simulink model "ProposedProblem1"  (R2013a)
settings: Solver=ode45  StartTime=0.0  StopTime=10.0  RelTol=1e-3
undefined symbols (not defined in the file): des, gcbh
settings Model: Creator=gabig  LastModifiedBy=gabig

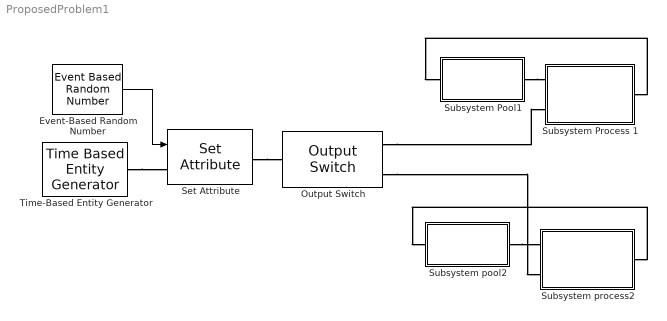
== system ProposedProblem1 ==
  Event-Based Random Number : EventBasedRandomNumber  Distribution=Arbitrary discrete  valueVecDisc=[1 2]  probVecDisc=[0.4 0.6]  Seed=12346
  Output Switch : OutputSwitch  NumberOutputPorts=2  SwitchingCriterion=From attribute  AttributeName=Type
  Set Attribute : SetAttribute  AttributeName=Type  AttributeFrom=Signal port  EvaluatedAttributeValue={ []}
  Subsystem Pool1 : Subsystem
  "Subsystem Process 1 " : Subsystem
  "Subsystem pool2 " : Subsystem
  "Subsystem process2 " : Subsystem
  Time-Based Entity Generator : TimeBasedEntityGenerator  Distribution=Uniform  Minimum=0.01  Maximum=0.2
  wires:
  Event-Based Random Number/1 -> Set Attribute/1
  connections:
  "Subsystem process2 "/RConn1 -- "Subsystem pool2 "/LConn1
  Time-Based Entity Generator/RConn1 -- Set Attribute/LConn1
  "Subsystem pool2 "/RConn1 -- "Subsystem process2 "/LConn1
  Output Switch/RConn2 -- "Subsystem process2 "/LConn2
  "Subsystem Process 1 "/RConn1 -- Subsystem Pool1/LConn1
  Output Switch/RConn1 -- "Subsystem Process 1 "/LConn2
  Set Attribute/RConn1 -- Output Switch/LConn1
  Subsystem Pool1/RConn1 -- "Subsystem Process 1 "/LConn1

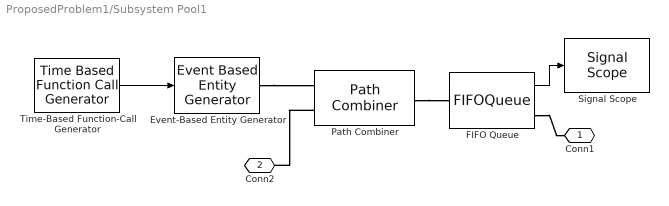
== system ProposedProblem1/Subsystem Pool1 ==
  Event-Based Entity Generator : EventBasedEntityGenerator  GenerateEntitiesUpon=Function call from port fcn
  FIFO Queue : FIFOQueue  Capacity=4  StatNumberInBlock=on
      settings: OutputPortMap=o1
  Path Combiner : PathCombiner  NumberInputPorts=2
  Signal Scope : SignalScope  LoadFcn=des.scope.CallbackSupport('seLoadFcn',gcbh)  StartFcn=des.scope.CallbackSupport('seStartFcn',gcbh)  StopFcn=des.scope.CallbackSupport('seStopFcn',gcbh)
      settings: CopyFcn=des.scope.CallbackSupport('seCopyFcn',gcbh)  DeleteFcn=des.scope.CallbackSupport('seDeleteFcn',gcbh)  PreSaveFcn=des.scope.CallbackSupport('sePreSaveFcn',gcbh)  NameChangeFcn=des.scope.CallbackSupport('seNameChangeFcn',gcbh)  OpenFcn=des.scope.CallbackSupport('seOpenFcn',gcbh)
  Time-Based Function-Call Generator : TimeBasedFunctionCallGenerator
  Conn1 : PMIOPort  Port=1  Side=Right
  "Conn2 " : PMIOPort  Port=2  Side=Left
  wires:
  FIFO Queue/1 -> Signal Scope/1
  Time-Based Function-Call Generator/1 -> Event-Based Entity Generator/1
  connections:
  Path Combiner/RConn1 -- FIFO Queue/LConn1
  Event-Based Entity Generator/RConn1 -- Path Combiner/LConn1
  Path Combiner/LConn2 -- "Conn2 "/RConn1
  FIFO Queue/RConn1 -- Conn1/RConn1

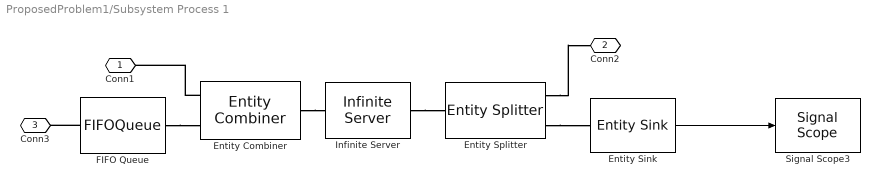
== system ProposedProblem1/Subsystem Process 1  ==
  Entity Combiner : EntityCombiner  NumberInputPorts=2
  Entity Sink : EntitySink  StatNumberArrived=on
  Entity Splitter : EntitySplitter  NumberOutputPorts=2
  FIFO Queue : FIFOQueue
  Infinite Server : InfiniteServer  ServiceTime=2
  Signal Scope3 : SignalScope  LoadFcn=des.scope.CallbackSupport('seLoadFcn',gcbh)  StartFcn=des.scope.CallbackSupport('seStartFcn',gcbh)  StopFcn=des.scope.CallbackSupport('seStopFcn',gcbh)
      settings: CopyFcn=des.scope.CallbackSupport('seCopyFcn',gcbh)  DeleteFcn=des.scope.CallbackSupport('seDeleteFcn',gcbh)  PreSaveFcn=des.scope.CallbackSupport('sePreSaveFcn',gcbh)  NameChangeFcn=des.scope.CallbackSupport('seNameChangeFcn',gcbh)  OpenFcn=des.scope.CallbackSupport('seOpenFcn',gcbh)
  Conn1 : PMIOPort  Port=1  Side=Left
  Conn2 : PMIOPort  Port=2  Side=Right
  Conn3 : PMIOPort  Port=3  Side=Left
  wires:
  Entity Sink/1 -> Signal Scope3/1
  connections:
  Infinite Server/RConn1 -- Entity Splitter/LConn1
  FIFO Queue/LConn1 -- Conn3/RConn1
  Entity Splitter/RConn1 -- Conn2/RConn1
  Entity Combiner/LConn1 -- Conn1/RConn1
  FIFO Queue/RConn1 -- Entity Combiner/LConn2
  Entity Splitter/RConn2 -- Entity Sink/LConn1
  Entity Combiner/RConn1 -- Infinite Server/LConn1

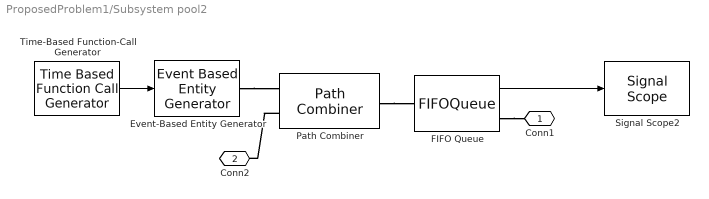
== system ProposedProblem1/Subsystem pool2  ==
  Event-Based Entity Generator : EventBasedEntityGenerator  GenerateEntitiesUpon=Function call from port fcn
  FIFO Queue : FIFOQueue  Capacity=8  StatNumberInBlock=on
      settings: OutputPortMap=o1
  Path Combiner : PathCombiner  NumberInputPorts=2
  Signal Scope2 : SignalScope  LoadFcn=des.scope.CallbackSupport('seLoadFcn',gcbh)  StartFcn=des.scope.CallbackSupport('seStartFcn',gcbh)  StopFcn=des.scope.CallbackSupport('seStopFcn',gcbh)
      settings: CopyFcn=des.scope.CallbackSupport('seCopyFcn',gcbh)  DeleteFcn=des.scope.CallbackSupport('seDeleteFcn',gcbh)  PreSaveFcn=des.scope.CallbackSupport('sePreSaveFcn',gcbh)  NameChangeFcn=des.scope.CallbackSupport('seNameChangeFcn',gcbh)  OpenFcn=des.scope.CallbackSupport('seOpenFcn',gcbh)
  Time-Based Function-Call Generator : TimeBasedFunctionCallGenerator
  Conn1 : PMIOPort  Port=1  Side=Right
  "Conn2 " : PMIOPort  Port=2  Side=Left
  wires:
  FIFO Queue/1 -> Signal Scope2/1
  Time-Based Function-Call Generator/1 -> Event-Based Entity Generator/1
  connections:
  Path Combiner/RConn1 -- FIFO Queue/LConn1
  Path Combiner/LConn2 -- "Conn2 "/RConn1
  FIFO Queue/RConn1 -- Conn1/RConn1
  Event-Based Entity Generator/RConn1 -- Path Combiner/LConn1

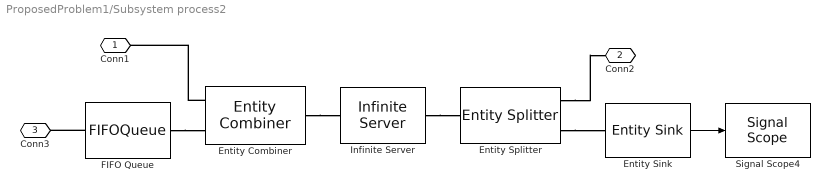
== system ProposedProblem1/Subsystem process2  ==
  Entity Combiner : EntityCombiner  NumberInputPorts=2
  Entity Sink : EntitySink  StatNumberArrived=on
  Entity Splitter : EntitySplitter  NumberOutputPorts=2
  FIFO Queue : FIFOQueue
  Infinite Server : InfiniteServer  ServiceTime=3
  Signal Scope4 : SignalScope  LoadFcn=des.scope.CallbackSupport('seLoadFcn',gcbh)  StartFcn=des.scope.CallbackSupport('seStartFcn',gcbh)  StopFcn=des.scope.CallbackSupport('seStopFcn',gcbh)
      settings: CopyFcn=des.scope.CallbackSupport('seCopyFcn',gcbh)  DeleteFcn=des.scope.CallbackSupport('seDeleteFcn',gcbh)  PreSaveFcn=des.scope.CallbackSupport('sePreSaveFcn',gcbh)  NameChangeFcn=des.scope.CallbackSupport('seNameChangeFcn',gcbh)  OpenFcn=des.scope.CallbackSupport('seOpenFcn',gcbh)
  Conn1 : PMIOPort  Port=1  Side=Left
  Conn2 : PMIOPort  Port=2  Side=Right
  Conn3 : PMIOPort  Port=3  Side=Left
  wires:
  Entity Sink/1 -> Signal Scope4/1
  connections:
  Entity Combiner/RConn1 -- Infinite Server/LConn1
  FIFO Queue/LConn1 -- Conn3/RConn1
  Entity Splitter/RConn1 -- Conn2/RConn1
  Entity Combiner/LConn1 -- Conn1/RConn1
  Infinite Server/RConn1 -- Entity Splitter/LConn1
  Entity Splitter/RConn2 -- Entity Sink/LConn1
  FIFO Queue/RConn1 -- Entity Combiner/LConn2
